simulink model "kf"  (R2019b)
settings: Solver=ode4  StartTime=0.0  StopTime=inf  FixedStep=0.05  RelTol=1e-3  EnableMultiTasking=on
libraries: robotlib x5
settings Model: Creator=ece446  LastModifiedBy=ivory
settings DataIOCC: ReturnWorkspaceOutputs=off
settings OptimizationCC: LifeSpan=Inf  MaxStackSize=64  EfficientTunableParamExpr=on
settings DebuggingCC: SFUnexpectedBacktrackingDiag=warning  SFNoUnconditionalDefaultTransitionDiag=warning  ArithmeticOperatorsInVariantConditions=warning
settings HardwareCC: ProdBitPerPointer=32  ProdBitPerSizeT=32  ProdBitPerPtrDiffT=32  ProdLargestAtomicFloat=None  ProdIntDivRoundTo=Undefined  ProdEndianess=Unspecified  ProdWordSize=32  ProdHWDeviceType=Generic->Unspecified (assume 32-bit Generic)
settings SFSimCC: SimUseLocalCustomCode=off  MATLABDynamicMemAlloc=off  CustomCodeUndefinedFunction=UseInterfaceOnly
settings RTWCC: SystemTargetFile=ert.tlc  HardwareBoard=Robot Operating System (ROS)  TLCOptions=-aInlineSetEventsForThisBaseRateFcn=TLC_FALSE -aSuppressMultiTaskScheduler=TLC_FALSE -aRateBasedStepFcn=0  TemplateMakefile=ert_default_tmf  GenerateReport=on  RTWUseLocalCustomCode=off  Toolchain=Catkin  IncludeHyperlinkInReport=on  LaunchReport=on  TargetLang=C++  GenerateTraceInfo=on  GenerateTraceReport=on  GenerateTraceReportSl=on  GenerateTraceReportSf=on  GenerateTraceReportEml=on
settings CodeAppCC: ForceParamTrailComments=on  IgnoreCustomStorageClasses=off  OperatorAnnotations=on  SimulinkDataObjDesc=on  SFDataObjDesc=on  MATLABFcnDesc=on  InsertBlockDesc=on  StateflowObjectComments=on  MATLABSourceComments=on
settings ERTTargetCC: MultiwordLength=2048  SupportContinuousTime=on
settings ConfigComp: CovMetricSettings=dw  CovHtmlReporting=on  CovSaveCumulativeToWorkspaceVar=on  CovSaveSingleToWorkspaceVar=on  CovExternalEMLEnable=off

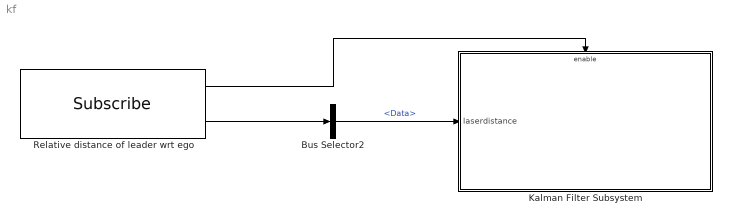
== system kf ==
  Bus Selector2 : BusSelector  OutputSignals=Data
  Kalman Filter Subsystem : Subsystem
  Relative distance of leader wrt ego : robotlib/Subscribe  topicSource=Specify your own  topic=d_relative  messageType=std_msgs/Float64  sampleTime=-1  messageQueueLength=1
      settings: SourceProductName=ROS Toolbox
  wires:
  Relative distance of leader wrt ego/2 -> Bus Selector2/1
  Bus Selector2/1 -> Kalman Filter Subsystem/1(laserdistance)  "<Data>"
  Relative distance of leader wrt ego/1 -> Kalman Filter Subsystem/Enable

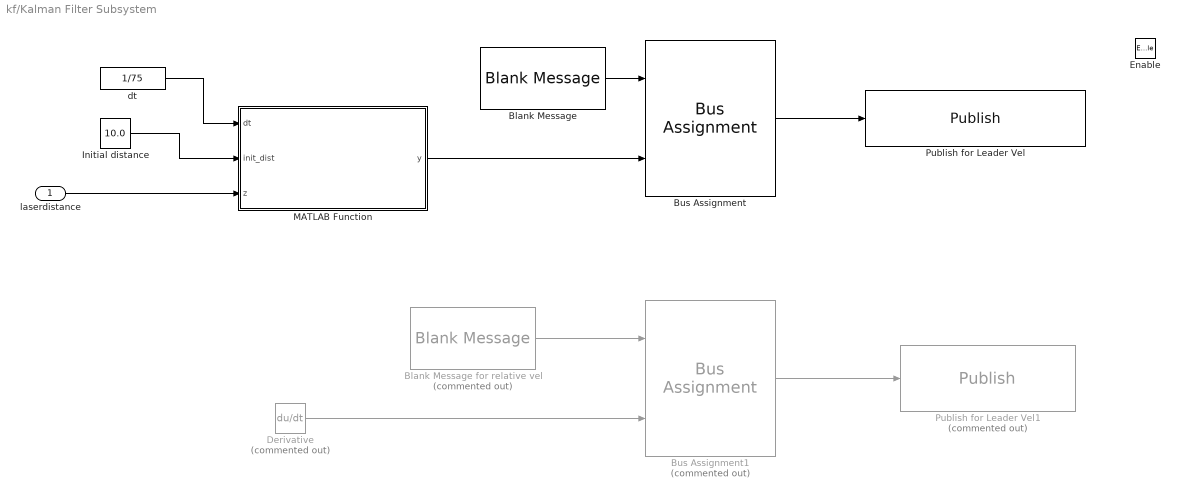
== system kf/Kalman Filter Subsystem ==
  laserdistance : Inport
  Enable : EnablePort
  Blank Message : robotlib/Blank Message  messageClass=Message  entityType=std_msgs/Float64  messageType=std_msgs/Float64  SampleTime=inf
      settings: SourceProductName=ROS Toolbox
  Blank Message for relative vel : robotlib/Blank Message  Commented=on  messageClass=Message  entityType=std_msgs/Float64  messageType=std_msgs/Float64  SampleTime=inf
      settings: SourceProductName=ROS Toolbox
  Bus Assignment : BusAssignment  AssignedSignals=Data
  Bus Assignment1 : BusAssignment  Commented=on  AssignedSignals=Data
  Derivative : Derivative  Commented=on  CoefficientInTFapproximation=0
  Initial distance : Constant  Value=10.0
  MATLAB Function : MATLAB Function  TreatAsAtomicUnit=on
  Publish for Leader Vel : robotlib/Publish  topicSource=Specify your own  topic=kf/dist  messageType=std_msgs/Float64  messageQueueLength=1
      settings: SourceProductName=ROS Toolbox
  Publish for Leader Vel1 : robotlib/Publish  Commented=on  topicSource=Specify your own  topic=/kalmanFilter/vel  messageType=std_msgs/Float32  messageQueueLength=1
      settings: SourceProductName=ROS Toolbox
  dt : Constant  Value=1/75
  wires:
  dt/1 -> MATLAB Function/1(dt)
  Initial distance/1 -> MATLAB Function/2(init_dist)
  Blank Message/1 -> Bus Assignment/1
  Blank Message for relative vel/1 -> Bus Assignment1/1
  Derivative/1 -> Bus Assignment1/2
  MATLAB Function/1(y) -> Bus Assignment/2
  Bus Assignment/1 -> Publish for Leader Vel/1
  Bus Assignment1/1 -> Publish for Leader Vel1/1
  laserdistance/1 -> MATLAB Function/3(z)

== matlab function kf/Kalman Filter Subsystem/MATLAB Function ==
  data: dt input; init_dist input; z input; y output
function y = kalmanfilter_dist(dt, init_dist, z) 
%#codegen

    % Initialize state transition matrix
    A=[ 1 dt 0;...     % [x  ]
        0 1 dt;...   ,,,,,  % [Vx]
        0 0 1];...     % [Ax]

    H = [init_dist 0 0];    % Initialize measurement matrix
    Q = eye(3);
    R = 1000 * eye(1);
    persistent x_est p_est z_old cnt             % Initial state conditions
    if isempty(x_est)
        x_est = zeros(3, 1);             % x_est=[x, Vx, Ax]'
        p_est = zeros(3, 3);
    end
    if isempty(cnt)
        cnt = 1;
    else
        cnt = cnt + 1;
    end

    if isempty(z_old)
        z_old = 10.0;
    end

    if (cnt <=50)
        z_old = z;
        x_prd = A * x_est;
        p_prd = A * p_est * A' + Q;
        % Estimation
        S = H * p_prd' * H' + R;
        B = H * p_prd';
        klm_gain = (S \ B)';
        % Estimated state and covariance
        x_est = x_prd + klm_gain * (z - H * x_prd);
        p_est = p_prd - klm_gain * H * p_prd;
        y = z_old;
    else
        if (z >= 80.0)
            z = z_old*0.98;
            if (z <= 10.0)
                z = 10.0;
            end
        end
        z_old = z;
        % Predicted state and covariance
        x_prd = A * x_est;
        p_prd = A * p_est * A' + Q;
        % Estimation
        S = H * p_prd' * H' + R;
        B = H * p_prd';
        klm_gain = (S \ B)';
        % Estimated state and covariance
        x_est = x_prd + klm_gain * (z - H * x_prd);
        p_est = p_prd - klm_gain * H * p_prd;
        % Compute the estimated measurements
    y = H * x_est;
    end
end                % of the function
